simulink model "spc63"  (R2020b)
settings: Solver=VariableStepAuto  StartTime=0.0  StopTime=tk2  RelTol=1e-3
values from neighbouring files (symbols this model uses):
  a = 8    [SPC_LAB6.m]
  b = 11    [SPC_LAB6.m]
  c = 2    [SPC_LAB6.m]
  steptime = 1    [SPC_LAB6.m]
  y = 3    [SPC_LAB6.m]
  y0 = 0    [SPC_LAB6.m]
undefined symbols (not defined in the file or in its folder): sigbuilder_block
libraries: pid_lib x2
settings Model: Creator=Konrad  LastModifiedBy=Konrad

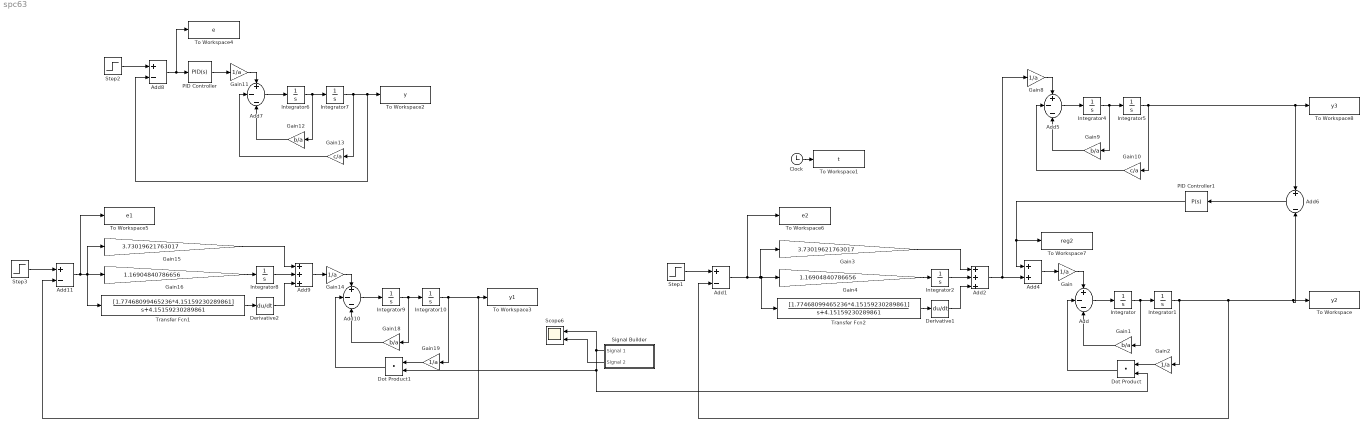
== system spc63 ==
  Add{,5,7,10} (4 alike) : Sum  Inputs=+--
  Add{1,6,8,11} (4 alike) : Sum  Inputs=+-
  Add2 : Sum  Inputs=+++
  Add4 : Sum
  Add9 : Sum  Inputs=+++
  Clock : Clock
  Derivative1 : Derivative
  Derivative2 : Derivative
  Dot Product : DotProduct  InputSameDT=on  OutDataTypeStr=Inherit: Inherit via internal rule
  Dot Product1 : DotProduct  InputSameDT=on  OutDataTypeStr=Inherit: Inherit via internal rule
  Gain{,2,8,11,14,19} (6 alike) : Gain  Gain=1/a
  Gain{1,9,12,18} (4 alike) : Gain  Gain=b/a
  Gain10 : Gain  Gain=c/a
  Gain13 : Gain  Gain=c/a
  Gain15 : Gain  Gain=3.73019621763017
  Gain16 : Gain  Gain=1.16904840786656
  Gain3 : Gain  Gain=3.73019621763017
  Gain4 : Gain  Gain=1.16904840786656
  Integrator{,1..2,4..10} (10 alike) : Integrator
  PID Controller : pid_lib/PID Controller  Controller=PID  Form=Parallel  TimeDomain=Continuous-time  UseExternalTs=off  SampleTime=-1  IntegratorMethod=Forward Euler  FilterMethod=Forward Euler  ControllerParametersSource=internal  P=3.73019621763017  I=1.16904840786656  D=1.77468099465236  UseFilter=on  N=4.15159230289861  TunerSelectOption=Transfer Function Based (PID Tuner App)  InitialConditionSource=internal  InitialConditionForIntegrator=0  InitialConditionForFilter=0  DifferentiatorICPrevScaledInput=0  ExternalReset=none  TrackingMode=off  Kt=1  LimitOutput=off  SatLimitsSource=internal  UpperSaturationLimit=inf  LowerSaturationLimit=-inf  LinearizeAsGain=on  AntiWindupMode=none  Kb=1  POutMin=[]  POutMax=[]  IOutMin=[]  IOutMax=[]  DOutMin=[]  DOutMax=[]  NOutMin=[]  NOutMax=[]  SumOutMin=[]  SumOutMax=[]  SaturationOutMin=[]  SaturationOutMax=[]  PParamMin=[]  PParamMax=[]  IParamMin=[]  IParamMax=[]  DParamMin=[]  DParamMax=[]  NParamMin=[]  NParamMax=[]  KbParamMin=[]  KbParamMax=[]  KtParamMin=[]  KtParamMax=[]  KbOutMin=[]  KbOutMax=[]  KtOutMin=[]  KtOutMax=[]  IntegratorOutMin=[]  IntegratorOutMax=[]  FilterOutMin=[]  FilterOutMax=[]  SumI1OutMin=[]  SumI1OutMax=[]  SumI2OutMin=[]  SumI2OutMax=[]  SumI3OutMin=[]  SumI3OutMax=[]  SumI4OutMin=[]  SumI4OutMax=[]  SumDOutMin=[]  SumDOutMax=[]  DifferentiatorOutMin=[]  DifferentiatorOutMax=[]  FilterDiffOutCoefMin=[]  FilterDiffOutCoefMax=[]  ReciprocalOutMin=[]  ReciprocalOutMax=[]  SumDenOutMin=[]  SumDenOutMax=[]  SumNumOutMin=[]  SumNumOutMax=[]  DivideOutMin=[]  DivideOutMax=[]  UdiffTsProdOutMin=[]  UdiffTsProdOutMax=[]  NTsProdOutMin=[]  NTsProdOutMax=[]  UintegralTsProdOutMin=[]  UintegralTsProdOutMax=[]  UngainTsProdOutMin=[]  UngainTsProdOutMax=[]  IntegratorContinuousStateAttributes=''  IntegratorStateMustResolveToSignalObject=off  IntegratorRTWStateStorageClass=Auto  FilterContinuousStateAttributes=''  FilterStateMustResolveToSignalObject=off  FilterRTWStateStorageClass=Auto  ParallelPVariant=InternalParameters  IdealPVariant=Disabled  IVariant=InternalParameters  DVariant=InternalParameters  IntegratorVariant=Continuous  SatVariant=Disabled  AWVariant=Passthrough  PCopyVariant=Disabled  TRVariant=Disabled  FdbkBlocksVariant=Forward  IdealPFdbkVariant=Disabled  SatFdbkVariant=Disabled  DerivativeFilterVariant=ContFilter  NVariant=InternalParameters  NCopyVariant=Disabled  FilterICVariant=InternalICsFilter  IntegratorICVariant=InternalICs  ExternalResetVariant=Disabled  TRSumVariant=Passthrough  SumFdbkVariant=Disabled  SumVariant=Sum_PID  TsampFilterVariant=InternalTs  TsampNgainVariant=Passthrough  TsampIntegralVariant=Passthrough  ExternalSaturationOutDataTypeStr=Inherit: Same as second input
  PID Controller1 : pid_lib/PID Controller  Controller=P  Form=Parallel  TimeDomain=Continuous-time  UseExternalTs=off  SampleTime=-1  IntegratorMethod=Forward Euler  FilterMethod=Forward Euler  ControllerParametersSource=internal  P=13.1519478848043  I=1.11751486797287  D=3.83355014487749  UseFilter=on  N=97.1470014765273  TunerSelectOption=Transfer Function Based (PID Tuner App)  InitialConditionSource=internal  InitialConditionForIntegrator=0  InitialConditionForFilter=0  DifferentiatorICPrevScaledInput=0  ExternalReset=none  TrackingMode=off  Kt=1  LimitOutput=off  SatLimitsSource=internal  UpperSaturationLimit=inf  LowerSaturationLimit=-inf  LinearizeAsGain=on  AntiWindupMode=none  Kb=1  POutMin=[]  POutMax=[]  IOutMin=[]  IOutMax=[]  DOutMin=[]  DOutMax=[]  NOutMin=[]  NOutMax=[]  SumOutMin=[]  SumOutMax=[]  SaturationOutMin=[]  SaturationOutMax=[]  PParamMin=[]  PParamMax=[]  IParamMin=[]  IParamMax=[]  DParamMin=[]  DParamMax=[]  NParamMin=[]  NParamMax=[]  KbParamMin=[]  KbParamMax=[]  KtParamMin=[]  KtParamMax=[]  KbOutMin=[]  KbOutMax=[]  KtOutMin=[]  KtOutMax=[]  IntegratorOutMin=[]  IntegratorOutMax=[]  FilterOutMin=[]  FilterOutMax=[]  SumI1OutMin=[]  SumI1OutMax=[]  SumI2OutMin=[]  SumI2OutMax=[]  SumI3OutMin=[]  SumI3OutMax=[]  SumI4OutMin=[]  SumI4OutMax=[]  SumDOutMin=[]  SumDOutMax=[]  DifferentiatorOutMin=[]  DifferentiatorOutMax=[]  FilterDiffOutCoefMin=[]  FilterDiffOutCoefMax=[]  ReciprocalOutMin=[]  ReciprocalOutMax=[]  SumDenOutMin=[]  SumDenOutMax=[]  SumNumOutMin=[]  SumNumOutMax=[]  DivideOutMin=[]  DivideOutMax=[]  UdiffTsProdOutMin=[]  UdiffTsProdOutMax=[]  NTsProdOutMin=[]  NTsProdOutMax=[]  UintegralTsProdOutMin=[]  UintegralTsProdOutMax=[]  UngainTsProdOutMin=[]  UngainTsProdOutMax=[]  IntegratorContinuousStateAttributes=''  IntegratorStateMustResolveToSignalObject=off  IntegratorRTWStateStorageClass=Auto  FilterContinuousStateAttributes=''  FilterStateMustResolveToSignalObject=off  FilterRTWStateStorageClass=Auto  ParallelPVariant=InternalParameters  IdealPVariant=Disabled  IVariant=Disabled  DVariant=Disabled  IntegratorVariant=Disabled  SatVariant=Disabled  AWVariant=Disabled  PCopyVariant=Disabled  TRVariant=Disabled  FdbkBlocksVariant=Forward  IdealPFdbkVariant=Disabled  SatFdbkVariant=Disabled  DerivativeFilterVariant=Disabled  NVariant=Disabled  NCopyVariant=Disabled_SignalSpec  FilterICVariant=Disabled  IntegratorICVariant=Disabled  ExternalResetVariant=Disabled  TRSumVariant=Passthrough  SumFdbkVariant=Disabled  SumVariant=Passthrough_P  TsampFilterVariant=InternalTs  TsampNgainVariant=Passthrough  TsampIntegralVariant=Disabled_SignalSpec  ExternalSaturationOutDataTypeStr=Inherit: Same as second input
  Scope6 : Scope  NumInputPorts=2
  Signal Builder : Subsystem  Tag=STV Subsys  LoadFcn=sigbuilder_block('load');  StartFcn=sigbuilder_block('start');  StopFcn=sigbuilder_block('stop');  ClipboardFcn=sigbuilder_block('clipboard');  mask(Sigbuilder block){tuvar=[0:10]}
      mask help: Simulink:masks:SigbuilderBlock_MD
      mask init:
      | if ~strcmp(get_param(bdroot(gcbh),'SimulationStatus'),'stopped') tuvar = sigbuilder_block('maskInit'); end
      settings: CopyFcn=sigbuilder_block('copy');  DeleteFcn=sigbuilder_block('delete');  ModelCloseFcn=sigbuilder_block('modelClose');  PreSaveFcn=sigbuilder_block('preSave');  PauseFcn=sigbuilder_block('pause');  ContinueFcn=sigbuilder_block('continue');  NameChangeFcn=sigbuilder_block('namechange');  OpenFcn=sigbuilder_block('open',[6 30 1012.5 447.75 ]);  CloseFcn=sigbuilder_block('close');
      mask Display: plot(0, 0, 100, 100,[2, 2, 32, 32, 2], [68, 8, 8, 68, 68],[32, 2], [38, 38], [32, 19, 2],[53, 60, 44], [32, 17, 17, 2],[16, 16, 31, 31]);txt = getActiveGroup(gcbh);text(2, 100, txt,'verticalAlignment', 'top');
  Step1 : Step  Time=steptime  Before=y0  After=y  SampleTime=0
  Step2 : Step  Time=steptime  Before=y0  After=y  SampleTime=0
  Step3 : Step  Time=steptime  Before=y0  After=y  SampleTime=0
  To Workspace : ToWorkspace  VariableName=y2  SampleTime=-1
  To Workspace1 : ToWorkspace  VariableName=t  SampleTime=-1
  To Workspace2 : ToWorkspace  VariableName=y  SampleTime=-1
  To Workspace3 : ToWorkspace  VariableName=y1  SampleTime=-1
  To Workspace4 : ToWorkspace  VariableName=e  SampleTime=-1
  To Workspace5 : ToWorkspace  VariableName=e1  SampleTime=-1
  To Workspace6 : ToWorkspace  VariableName=e2  SampleTime=-1
  To Workspace7 : ToWorkspace  VariableName=reg2  SampleTime=-1
  To Workspace8 : ToWorkspace  VariableName=y3  SampleTime=-1
  Transfer Fcn1 : TransferFcn  Numerator=[1.77468099465236*4.15159230289861]  Denominator=[1 4.15159230289861]
  Transfer Fcn2 : TransferFcn  Numerator=[1.77468099465236*4.15159230289861]  Denominator=[1 4.15159230289861]
  wires:
  Gain/1 -> Add/1
  Add/1 -> Integrator/1
  Integrator/1 -> Integrator1/1, Gain1/1
  Gain1/1 -> Add/3
  Integrator1/1 -> Add1/2, Add6/2, To Workspace/1, Gain2/1
  Gain2/1 -> Dot Product/1
  Dot Product/1 -> Add/2
  Clock/1 -> To Workspace1/1
  Step1/1 -> Add1/1
  Add4/1 -> Gain/1
  Add2/1 -> Add4/2, Gain8/1
  Gain8/1 -> Add5/1
  Gain9/1 -> Add5/3
  Add5/1 -> Integrator4/1
  Gain10/1 -> Add5/2
  Integrator4/1 -> Integrator5/1, Gain9/1
  Integrator5/1 -> To Workspace8/1, Add6/1, Gain10/1
  Gain12/1 -> Add7/3
  Integrator7/1 -> Gain13/1, Add8/2, To Workspace2/1
  Integrator6/1 -> Integrator7/1, Gain12/1
  Gain11/1 -> Add7/1
  Add7/1 -> Integrator6/1
  Step2/1 -> Add8/1
  Gain13/1 -> Add7/2
  Step3/1 -> Add11/1
  Gain14/1 -> Add10/1
  Integrator9/1 -> Integrator10/1, Gain18/1
  Gain18/1 -> Add10/3
  Add10/1 -> Integrator9/1
  Integrator10/1 -> Gain19/1, Add11/2, To Workspace3/1
  Dot Product1/1 -> Add10/2
  Gain19/1 -> Dot Product1/1
  PID Controller/1 -> Gain11/1
  Add8/1 -> To Workspace4/1, PID Controller/1
  Add11/1 -> To Workspace5/1, Gain15/1, Transfer Fcn1/1, Gain16/1
  Derivative2/1 -> Add9/3
  Integrator8/1 -> Add9/2
  Transfer Fcn1/1 -> Derivative2/1
  Gain15/1 -> Add9/1
  Gain16/1 -> Integrator8/1
  Add9/1 -> Gain14/1
  Signal Builder/1(Signal 1) -> Dot Product/2, Dot Product1/2, Scope6/1
  Signal Builder/2(Signal 2) -> Scope6/2
  Add6/1 -> PID Controller1/1
  PID Controller1/1 -> Add4/1, To Workspace7/1
  Add1/1 -> Gain3/1, Transfer Fcn2/1, Gain4/1, To Workspace6/1
  Transfer Fcn2/1 -> Derivative1/1
  Gain4/1 -> Integrator2/1
  Integrator2/1 -> Add2/2
  Derivative1/1 -> Add2/3
  Gain3/1 -> Add2/1

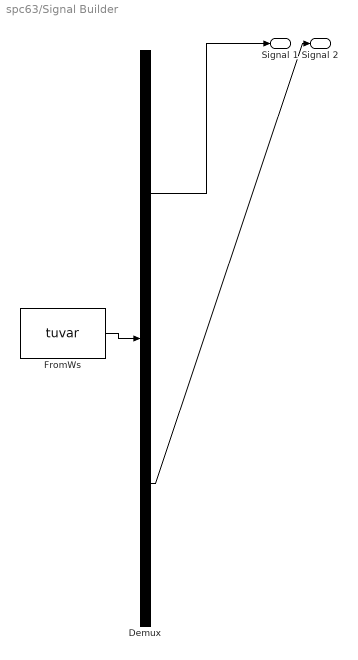
== system spc63/Signal Builder ==
  Demux : Demux  Tag=STV Demux  Outputs=2
      settings: DisplayOption=none
  FromWs : FromWorkspace  Tag=STV FromWs  VariableName=tuvar  OutputAfterFinalValue=Holding final value
      SigBuilderData=|
      | common.afterFinalStr = 'Hold final value'
      | common.sampleTime = '0'
      | dataSet.timeRange = [0 30]
      | dataSet.name = 'Group 1'
      | sbobj.Groups.Name = 'Group 1'
      | sbobj.Groups.Signals(1).Name = 'Signal 1'
      | sbobj.Groups.Signals(1).XData = [0 6 26 30]
      | sbobj.Groups.Signals(1).YData = [2 2 3 3]
      | sbobj.Groups.Signals(2).Name = 'Signal 2'
      | sbobj.Groups.Signals(2).XData = [0 0.01 0.02 0.03 0.04 0.05 0.06 0.07 0.08 0.09 0.1 0.11 ... (3001 elements, 1x3001)]
      | sbobj.Groups.Signals(2).YData = [2.01986852431 2.01988091762 2.01989332638 2.01990575063 2.01991819038 2.01993064567 2.01994311653 2.01995560298 2.01996810506 2.01998062279 2.0199931562 2.02000570533 ... (3001 elements, 1x3001)]
      | sbobj.Groups.TimeRange = [0 30]
  Signal 1 : Outport  Tag=STV Outport
  Signal 2 : Outport  Tag=STV Outport  Port=2
  wires:
  FromWs/1 -> Demux/1
  Demux/1 -> Signal 1/1
  Demux/2 -> Signal 2/1
